simulink model "SPWM"  (R2020a)
settings: Solver=VariableStepAuto  StartTime=0.0  StopTime=10.0  RelTol=1e-3
model workspace (MAT data in the model file):
  C = 1e-06
  L = 0.001
  R = 20
  udc = 100
  w = 1
libraries: simulink x3
settings Model: Creator=ZhuanZ（无密码）  LastModifiedBy=ZhuanZ（无密码）

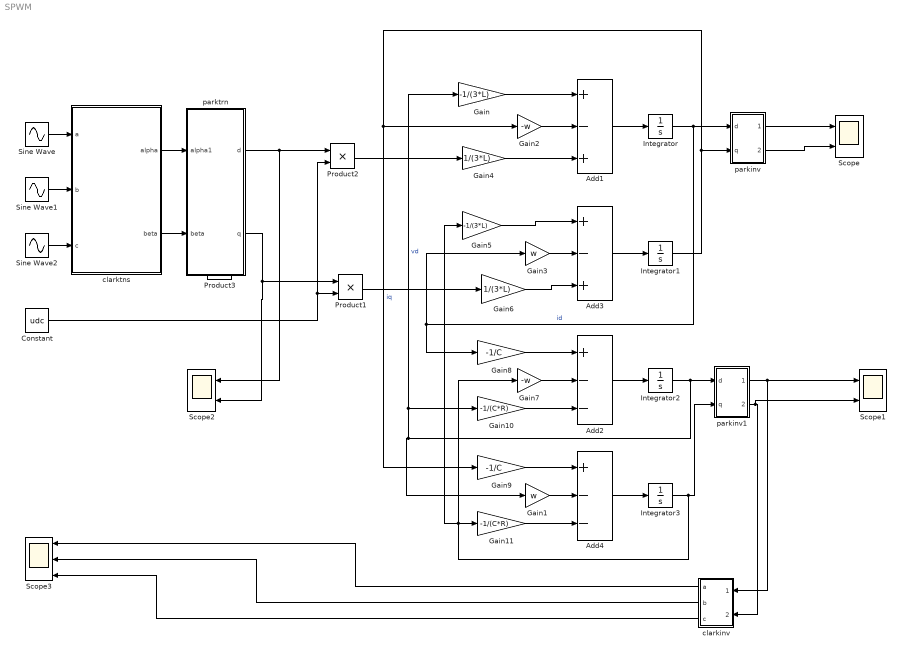
== system SPWM ==
  Add1 : Sum  Inputs=+-+
  Add2 : Sum  Inputs=+--
  Add3 : Sum  Inputs=+-+
  Add4 : Sum  Inputs=+--
  Constant : Constant  Value=udc
  Gain : Gain  Gain=-1/(3*L)
  Gain1 : Gain  Gain=w
  Gain10 : Gain  Gain=-1/(C*R)
  Gain11 : Gain  Gain=-1/(C*R)
  Gain2 : Gain  Gain=-w
  Gain3 : Gain  Gain=w
  Gain4 : Gain  Gain=1/(3*L)
  Gain5 : Gain  Gain=-1/(3*L)
  Gain6 : Gain  Gain=1/(3*L)
  Gain7 : Gain  Gain=-w
  Gain8 : Gain  Gain=-1/C
  Gain9 : Gain  Gain=-1/C
  Integrator{,1..3} (4 alike) : Integrator
  Product1 : Product  RndMeth=Zero
  Product2 : Product  RndMeth=Zero
  Product3 : Product  RndMeth=Zero
  Scope : Scope  NumInputPorts=2
  Scope1 : Scope  NumInputPorts=2
  Scope2 : Scope  NumInputPorts=2
  Scope3 : Scope  NumInputPorts=3
  Sine Wave : Sin  Frequency=2*pi*50  SampleTime=0
  Sine Wave1 : Sin  Frequency=2*pi*50  Phase=pi/3  SampleTime=0
  Sine Wave2 : Sin  Frequency=2*pi*50  Phase=2*pi/3  SampleTime=0
  clarkinv : Subsystem
  clarktns : Subsystem
  parkinv : Subsystem
  parkinv1 : Subsystem
  parktrn : Subsystem
  wires:
  Gain/1 -> Add1/1
  Gain2/1 -> Add1/2
  Gain4/1 -> Add1/3
  Gain5/1 -> Add3/1
  Gain6/1 -> Add3/3
  Gain3/1 -> Add3/2
  Product2/1 -> Gain4/1
  Add1/1 -> Integrator/1
  Add3/1 -> Integrator1/1
  Add2/1 -> Integrator2/1
  Add4/1 -> Integrator3/1
  Integrator3/1 -> Gain5/1, Gain7/1, Gain11/1, parkinv1/2(q)
  Gain1/1 -> Add4/2
  Gain7/1 -> Add2/2
  Gain8/1 -> Add2/1
  Gain9/1 -> Add4/1
  Gain10/1 -> Add2/3
  Gain11/1 -> Add4/3
  Sine Wave2/1 -> clarktns/3(c)
  Sine Wave1/1 -> clarktns/2(b)
  Sine Wave/1 -> clarktns/1(a)
  clarktns/1(alpha) -> parktrn/1(alpha1)
  clarktns/2(beta) -> parktrn/2(beta)
  parktrn/1(d) -> Scope2/1, Product2/1
  parktrn/2(q) -> Product1/1, Scope2/2
  Constant/1 -> Product2/2, Product1/2
  Integrator/1 -> Gain8/1, Gain3/1, parkinv/1(d)  "id"
  Integrator1/1 -> Gain2/1, Gain9/1, parkinv/2(q)  "iq"
  Integrator2/1 -> Gain10/1, Gain/1, Gain1/1, parkinv1/1(d)  "vd"
  parkinv1/1(alpha) -> Scope1/1, clarkinv/1(alpha)
  parkinv1/2(beta) -> Scope1/2, clarkinv/2(beta)
  parkinv/1(alpha) -> Scope/1
  parkinv/2(beta) -> Scope/2
  clarkinv/1(a) -> Scope3/1
  clarkinv/2(b) -> Scope3/2
  clarkinv/3(c) -> Scope3/3
  Product1/1 -> Gain6/1

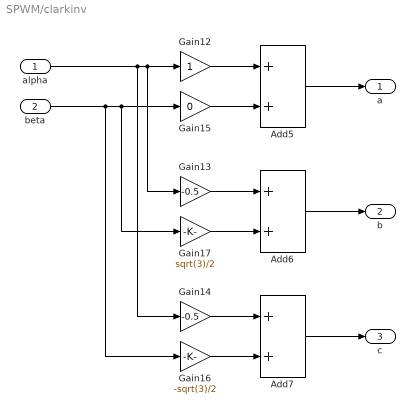
== system SPWM/clarkinv ==
  alpha : Inport
  beta : Inport  Port=2
  Add5 : Sum
  Add6 : Sum
  Add7 : Sum
  Gain12 : Gain
  Gain13 : Gain  Gain=-0.5
  Gain14 : Gain  Gain=-0.5
  Gain15 : Gain  Gain=0
  Gain16 : Gain  Gain=-sqrt(3)/2
  Gain17 : Gain  Gain=sqrt(3)/2
  a : Outport
  b : Outport  Port=2
  c : Outport  Port=3
  wires:
  Add5/1 -> a/1
  Gain13/1 -> Add6/1
  alpha/1 -> Gain14/1, Gain13/1, Gain12/1
  Gain16/1 -> Add7/2
  Gain14/1 -> Add7/1
  Add7/1 -> c/1
  Gain12/1 -> Add5/1
  Add6/1 -> b/1
  Gain17/1 -> Add6/2
  beta/1 -> Gain16/1, Gain17/1, Gain15/1
  Gain15/1 -> Add5/2

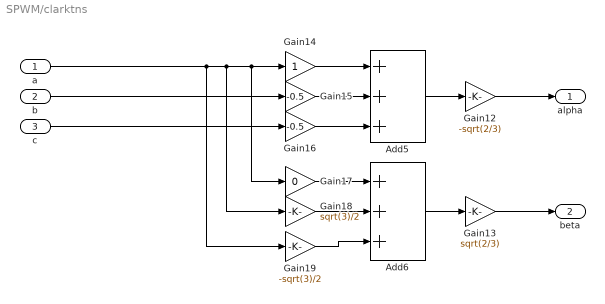
== system SPWM/clarktns ==
  a : Inport
  b : Inport  Port=2
  c : Inport  Port=3
  Add5 : Sum  Inputs=+++
  Add6 : Sum  Inputs=+++
  Gain12 : Gain  Gain=-sqrt(2/3)
  Gain13 : Gain  Gain=sqrt(2/3)
  Gain14 : Gain
  Gain15 : Gain  Gain=-0.5
  Gain16 : Gain  Gain=-0.5
  Gain17 : Gain  Gain=0
  Gain18 : Gain  Gain=sqrt(3)/2
  Gain19 : Gain  Gain=-sqrt(3)/2
  alpha : Outport
  beta : Outport  Port=2
  wires:
  Gain12/1 -> alpha/1
  Gain17/1 -> Add6/1
  a/1 -> Gain19/1, Gain18/1, Gain17/1, Gain14/1
  b/1 -> Gain15/1
  Gain18/1 -> Add6/2
  Gain19/1 -> Add6/3
  Gain14/1 -> Add5/1
  Add5/1 -> Gain12/1
  c/1 -> Gain16/1
  Add6/1 -> Gain13/1
  Gain13/1 -> beta/1
  Gain16/1 -> Add5/3
  Gain15/1 -> Add5/2

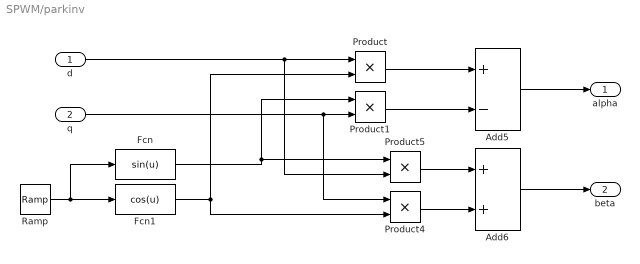
== system SPWM/parkinv ==
  d : Inport
  q : Inport  Port=2
  Add5 : Sum  Inputs=+-
  Add6 : Sum
  Fcn : Fcn  Expr=sin(u)
  Fcn1 : Fcn  Expr=cos(u)
  Product{,1,4..5} (4 alike) : Product  RndMeth=Zero
  Ramp : simulink/Sources/Ramp  slope=1  start=0  InitialOutput=0
  alpha : Outport
  beta : Outport  Port=2
  wires:
  q/1 -> Product4/1, Product1/2
  Add6/1 -> beta/1
  Fcn/1 -> Product1/1, Product5/1
  d/1 -> Product/1, Product5/2
  Product4/1 -> Add6/2
  Product/1 -> Add5/1
  Product1/1 -> Add5/2
  Fcn1/1 -> Product4/2, Product/2
  Product5/1 -> Add6/1
  Add5/1 -> alpha/1
  Ramp/1 -> Fcn1/1, Fcn/1

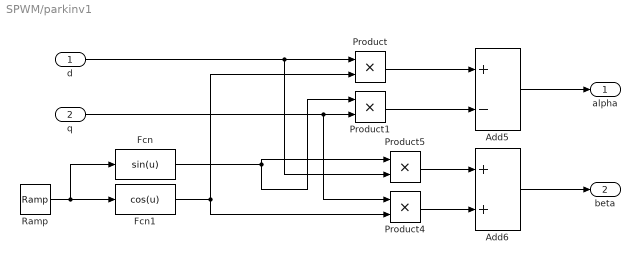
== system SPWM/parkinv1 ==
  d : Inport
  q : Inport  Port=2
  Add5 : Sum  Inputs=+-
  Add6 : Sum
  Fcn : Fcn  Expr=sin(u)
  Fcn1 : Fcn  Expr=cos(u)
  Product{,1,4..5} (4 alike) : Product  RndMeth=Zero
  Ramp : simulink/Sources/Ramp  slope=1  start=0  InitialOutput=0
  alpha : Outport
  beta : Outport  Port=2
  wires:
  q/1 -> Product4/1, Product1/2
  Add6/1 -> beta/1
  Fcn/1 -> Product1/1, Product5/1
  d/1 -> Product/1, Product5/2
  Product4/1 -> Add6/2
  Product/1 -> Add5/1
  Product1/1 -> Add5/2
  Fcn1/1 -> Product4/2, Product/2
  Product5/1 -> Add6/1
  Add5/1 -> alpha/1
  Ramp/1 -> Fcn1/1, Fcn/1

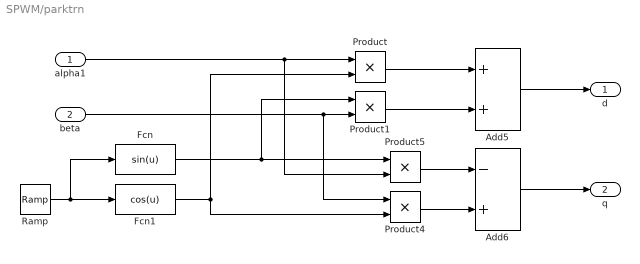
== system SPWM/parktrn ==
  alpha1 : Inport
  beta : Inport  Port=2
  Add5 : Sum
  Add6 : Sum  Inputs=-+
  Fcn : Fcn  Expr=sin(u)
  Fcn1 : Fcn  Expr=cos(u)
  Product{,1,4..5} (4 alike) : Product  RndMeth=Zero
  Ramp : simulink/Sources/Ramp  slope=1  start=0  InitialOutput=0
  d : Outport
  q : Outport  Port=2
  wires:
  Fcn1/1 -> Product4/2, Product/2
  alpha1/1 -> Product/1, Product5/2
  beta/1 -> Product4/1, Product1/2
  Product/1 -> Add5/1
  Add5/1 -> d/1
  Fcn/1 -> Product1/1, Product5/1
  Product4/1 -> Add6/2
  Product5/1 -> Add6/1
  Product1/1 -> Add5/2
  Add6/1 -> q/1
  Ramp/1 -> Fcn1/1, Fcn/1
